simulink model "session 8 page 72"  (R2021b)
settings: Solver=VariableStepAuto  StartTime=0.0  StopTime=10.0  RelTol=1e-3
settings Model: Creator=Pixle  LastModifiedBy=Pixle

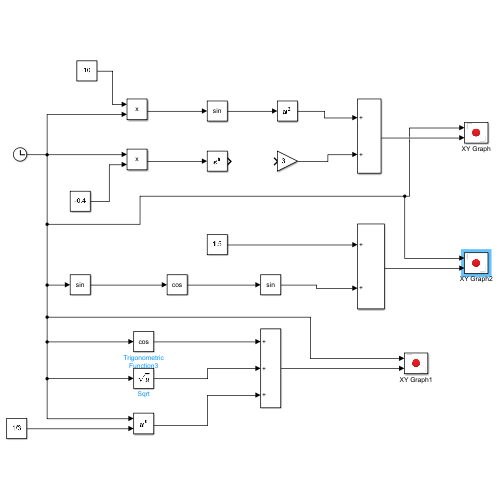
[thumbnail: Simulink's stored preview of the top-level diagram]
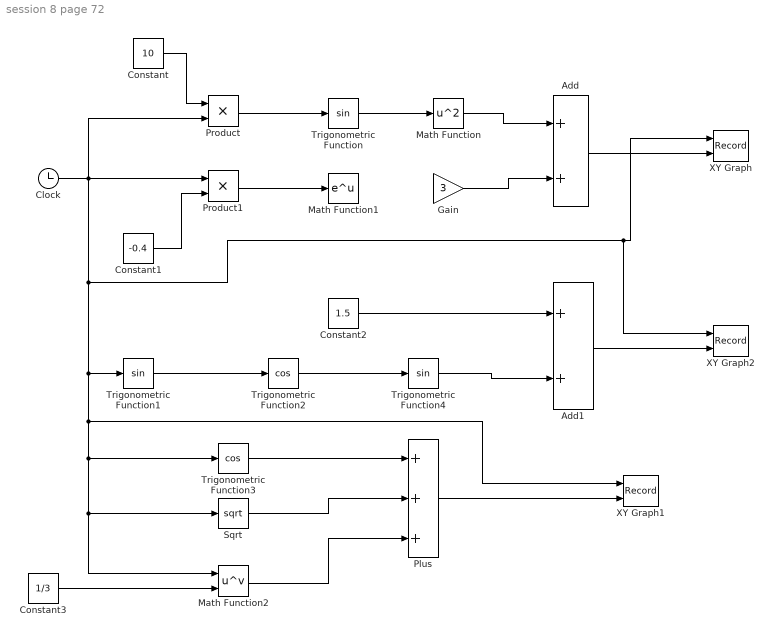
== system session 8 page 72 ==
  Add : Sum
  Add1 : Sum
  Clock : Clock
  Constant : Constant  Value=10
  Constant1 : Constant  Value=-0.4
  Constant2 : Constant  Value=1.5
  Constant3 : Constant  Value=1/3
  Gain : Gain  Gain=3
  Math Function : Math  Operator=square  SaturateOnIntegerOverflow=on
      settings: LockScale=on
  Math Function1 : Math  SaturateOnIntegerOverflow=on
  Math Function2 : Math  Operator=pow  SaturateOnIntegerOverflow=on
  Plus : Sum  Inputs=+++
  Product : Product
  Product1 : Product
  Sqrt : Sqrt  SaturateOnIntegerOverflow=on
  Trigonometric Function : Trigonometry
  Trigonometric Function1 : Trigonometry
  Trigonometric Function2 : Trigonometry  Operator=cos
  Trigonometric Function3 : Trigonometry  Operator=cos
  Trigonometric Function4 : Trigonometry
  XY Graph : Record  FileSettingsInternal="{\"entries\":[{\"content\":{\"excelSettings\":{\"content\":{},\"type\":\"Streamout.ExcelSettings\"}},\"type\":\"Streamout.FileSettingStorage\",\"uuid\":\"fdc99e3b-b4e1-4121-8778-01955f2c67a3\"}],\"packageUris\":[\"http://schema.mathworks.com/mf0/streamout_blocks/R2020a\"],\"version\":\"1.0\"}"  Layout=[1 1]  SignalsInternal="{\"entries\":[{\"content\":{\"signals\":[{\"content\":{\"blockPath\":[\"untitled/XY Graph\"],\"channel\":[],\"dimensions\":[1],\"domain\":\"untitled/XY Graph\",\"lineColor\":\"#a2142f\",\"plots\":[1],\"port\":1,\"sid\":[],\"signalID\":32,\"signalName\":\"XY Graph:1\"},\"type\":\"RecordBlkView.Signal\",\"uuid\":\"a47b6cd1-f629-454a-929b-723ab5bc6d17\"},{\"content\":{\"blockPath\":[\"untitled/XY Graph\"],\"channel\":[],\"dimensions\":[1],\"domain\":\"untitled/XY Graph\",\"lineColor\":\"#139fff\",\"plots\":[1],\"port\":2,\"sid\":[],\"signalID\":35,\"signalName\":\"XY Graph:2\"},\"type\":\"RecordBlkView.Signal\",\"uuid\":\"6d97634d-fde0-4a7e-97df-3c87e7fd1e99\"}]},\"type\":\"RecordBlkView.InputSignals\",\"uuid\":\"d6cd473c-ba3d-4c5c-bc3a-4031f16fcc4e\"}],\"packageUris\":[\"http://schema.mathworks.com/mf0/streamout_blocks/R2020a\"],\"version\":\"1.0\"}"  VisualizationBindings="{\"xyplotplugin\":{\"info\":[{\"series\":[{\"bindingParametersList\":[{\"parameter\":\"X-Axis\",\"signalID\":32,\"signalName\":\"XY Graph:1\"},{\"parameter\":\"Y-Axis\",\"signalID\":35,\"signalName\":\"XY Graph:2\"}],\"seriesID\":28368}],\"subplotID\":1}]}}"  CompatibilityTag=XY
  XY Graph1 : Record  FileSettingsInternal="{\"entries\":[{\"content\":{\"excelSettings\":{\"content\":{},\"type\":\"Streamout.ExcelSettings\"}},\"type\":\"Streamout.FileSettingStorage\",\"uuid\":\"d57c0f46-626b-4069-b607-cba39970bab8\"}],\"packageUris\":[\"http://schema.mathworks.com/mf0/streamout_blocks/R2020a\"],\"version\":\"1.0\"}"  Layout=[1 1]  SignalsInternal="{\"entries\":[{\"content\":{\"signals\":[{\"content\":{\"blockPath\":[\"untitled/XY Graph1\"],\"channel\":[],\"dimensions\":[1],\"domain\":\"untitled/XY Graph1\",\"lineColor\":\"#a2142f\",\"plots\":[1],\"port\":1,\"sid\":[],\"signalID\":40,\"signalName\":\"XY Graph:1\"},\"type\":\"RecordBlkView.Signal\",\"uuid\":\"667c1817-9e1c-4fc4-ade9-12a1d20023c0\"},{\"content\":{\"blockPath\":[\"untitled/XY Graph1\"],\"channel\":[],\"dimensions\":[1],\"domain\":\"untitled/XY Graph1\",\"lineColor\":\"#139fff\",\"plots\":[1],\"port\":2,\"sid\":[],\"signalID\":43,\"signalName\":\"XY Graph:2\"},\"type\":\"RecordBlkView.Signal\",\"uuid\":\"4412b04e-17f5-4e0f-a4b4-d7b1bd087fba\"}]},\"type\":\"RecordBlkView.InputSignals\",\"uuid\":\"ed243731-e088-46e2-91f8-cdc349b4cd8c\"}],\"packageUris\":[\"http://schema.mathworks.com/mf0/streamout_blocks/R2020a\"],\"version\":\"1.0\"}"  VisualizationBindings="{\"xyplotplugin\":{\"info\":[{\"series\":[{\"bindingParametersList\":[{\"parameter\":\"X-Axis\",\"signalID\":40,\"signalName\":\"XY Graph:1\"},{\"parameter\":\"Y-Axis\",\"signalID\":43,\"signalName\":\"XY Graph:2\"}],\"seriesID\":51599}],\"subplotID\":1}]}}"  CompatibilityTag=XY
  XY Graph2 : Record  FileSettingsInternal="{\"entries\":[{\"content\":{\"excelSettings\":{\"content\":{},\"type\":\"Streamout.ExcelSettings\"}},\"type\":\"Streamout.FileSettingStorage\",\"uuid\":\"07bc6ceb-9494-404f-a287-77032e226b16\"}],\"packageUris\":[\"http://schema.mathworks.com/mf0/streamout_blocks/R2020a\"],\"version\":\"1.0\"}"  Layout=[1 1]  SignalsInternal="{\"entries\":[{\"content\":{\"signals\":[{\"content\":{\"blockPath\":[\"untitled/XY Graph2\"],\"channel\":[],\"dimensions\":[1],\"domain\":\"untitled/XY Graph2\",\"lineColor\":\"#a2142f\",\"plots\":[1],\"port\":1,\"sid\":[],\"signalID\":48,\"signalName\":\"XY Graph:1\"},\"type\":\"RecordBlkView.Signal\",\"uuid\":\"d1ce5b06-d41b-429a-b48d-3e98f0234a9e\"},{\"content\":{\"blockPath\":[\"untitled/XY Graph2\"],\"channel\":[],\"dimensions\":[1],\"domain\":\"untitled/XY Graph2\",\"lineColor\":\"#139fff\",\"plots\":[1],\"port\":2,\"sid\":[],\"signalID\":51,\"signalName\":\"XY Graph:2\"},\"type\":\"RecordBlkView.Signal\",\"uuid\":\"a7397a2d-dc75-4263-a1d6-ef82811891f3\"}]},\"type\":\"RecordBlkView.InputSignals\",\"uuid\":\"f12b0ce8-8241-4b11-abd7-485405d525ec\"}],\"packageUris\":[\"http://schema.mathworks.com/mf0/streamout_blocks/R2020a\"],\"version\":\"1.0\"}"  VisualizationBindings="{\"xyplotplugin\":{\"info\":[{\"series\":[{\"bindingParametersList\":[{\"parameter\":\"X-Axis\",\"signalID\":48,\"signalName\":\"XY Graph:1\"},{\"parameter\":\"Y-Axis\",\"signalID\":51,\"signalName\":\"XY Graph:2\"}],\"seriesID\":11060}],\"subplotID\":1}]}}"  CompatibilityTag=XY
  wires:
  Constant/1 -> Product/1
  Product/1 -> Trigonometric Function/1
  Trigonometric Function/1 -> Math Function/1
  Constant1/1 -> Product1/2
  Product1/1 -> Math Function1/1
  Math Function/1 -> Add/1
  Gain/1 -> Add/2
  Add/1 -> XY Graph/2
  Constant2/1 -> Add1/1
  Trigonometric Function4/1 -> Add1/2
  Trigonometric Function2/1 -> Trigonometric Function4/1
  Trigonometric Function1/1 -> Trigonometric Function2/1
  Constant3/1 -> Math Function2/2
  Math Function2/1 -> Plus/3
  Sqrt/1 -> Plus/2
  Trigonometric Function3/1 -> Plus/1
  Plus/1 -> XY Graph1/2
  Add1/1 -> XY Graph2/2
  Clock/1 -> Product/2, XY Graph2/1, XY Graph/1, Trigonometric Function1/1, XY Graph1/1, Trigonometric Function3/1, Sqrt/1, Math Function2/1, Product1/1
